simulink model "ClosedLoop_CqCsc"  (R2023b)
settings: Solver=VariableStepAuto  StartTime=0.0  StopTime=10.0  RelTol=1e-6
libraries: cstblocks x4
settings Model: Creator=randolf  LastModifiedBy=randolf

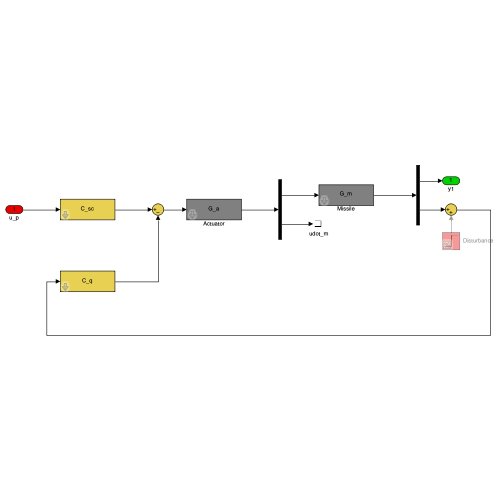
[thumbnail: Simulink's stored preview of the top-level diagram]
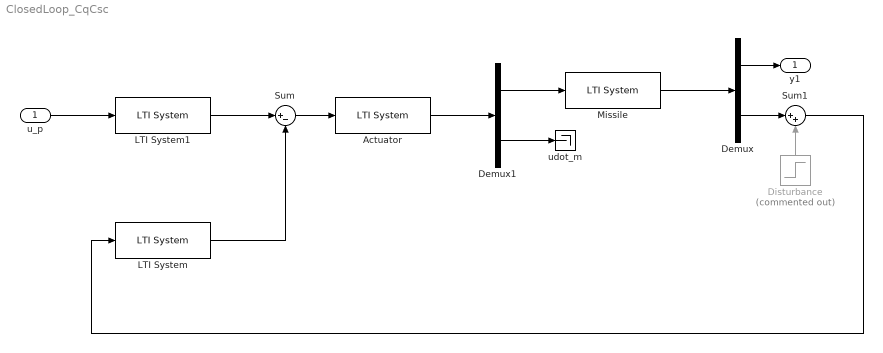
== system ClosedLoop_CqCsc ==
  u_p : Inport
  Actuator : cstblocks/LTI System  sys=G_a  IC=[]  PadeOrder=0
  Demux : Demux  Outputs=2
  Demux1 : Demux  Outputs=2
  Disturbance : Step  Commented=on  SampleTime=0
  LTI System : cstblocks/LTI System  sys=C_q  IC=[]  PadeOrder=0
  LTI System1 : cstblocks/LTI System  sys=C_sc  IC=[]  PadeOrder=0
  Missile : cstblocks/LTI System  sys=G_m  IC=[]  PadeOrder=0
  Sum : Sum  Inputs=|+-
  Sum1 : Sum  Inputs=|++
  udot_m : Terminator
  y1 : Outport
  wires:
  Demux1/1 -> Missile/1
  LTI System/1 -> Sum/2
  Demux1/2 -> udot_m/1
  Missile/1 -> Demux/1
  Actuator/1 -> Demux1/1
  Sum/1 -> Actuator/1
  Demux/1 -> y1/1
  LTI System1/1 -> Sum/1
  Demux/2 -> Sum1/1
  Sum1/1 -> LTI System/1
  Disturbance/1 -> Sum1/2
  u_p/1 -> LTI System1/1
